simulink model "dft_laplace_and_divided_by_GSFR"  (R2019b)
settings: Solver=VariableStepAuto  StartTime=0.0  StopTime=20  RelTol=1e-3
settings Model: Creator=ruiva  LastModifiedBy=ruiva

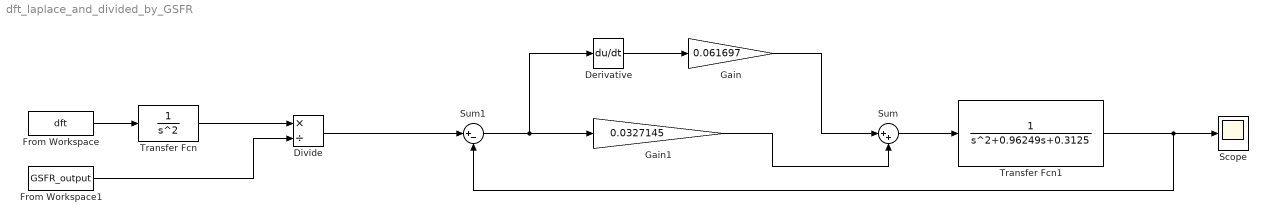
== system dft_laplace_and_divided_by_GSFR ==
  Derivative : Derivative
  Divide : Product  Inputs=*/
  From Workspace : FromWorkspace  VariableName=dft  SampleTime=0
  From Workspace1 : FromWorkspace  VariableName=GSFR_output  SampleTime=0
  Gain : Gain  Gain=0.061697
  Gain1 : Gain  Gain=0.0327145
  Scope : Scope
  Sum : Sum  Inputs=|++
  Sum1 : Sum  Inputs=|+-
  Transfer Fcn : TransferFcn  Denominator=[1 0 0]
  Transfer Fcn1 : TransferFcn  Denominator=[1 0.96249 0.3125]
  wires:
  From Workspace/1 -> Transfer Fcn/1
  Transfer Fcn/1 -> Divide/1
  From Workspace1/1 -> Divide/2
  Divide/1 -> Sum1/1
  Derivative/1 -> Gain/1
  Gain/1 -> Sum/1
  Gain1/1 -> Sum/2
  Sum1/1 -> Derivative/1, Gain1/1
  Sum/1 -> Transfer Fcn1/1
  Transfer Fcn1/1 -> Sum1/2, Scope/1
